simulink model "SARADC"  (R2024a)
settings: Solver=VariableStepAuto  StartTime=0.0  StopTime=10.0  RelTol=1e-3
undefined symbols (not defined in the file): bs2, bs3, bs4, bs5, thnoise_samp
settings Model: Creator=sjtu  LastModifiedBy=sjtu

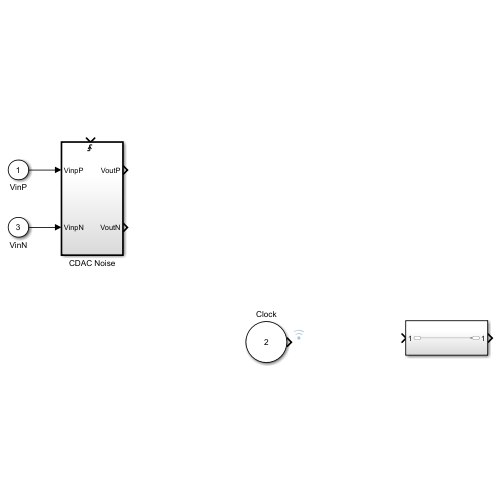
[thumbnail: Simulink's stored preview of the top-level diagram]
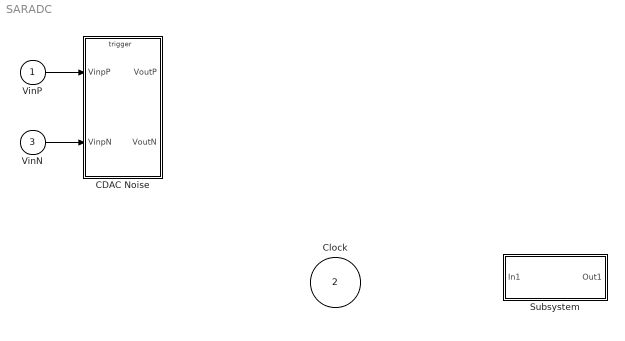
== system SARADC ==
  VinP : Inport
  Clock : Inport  Port=2
  VinN : Inport  Port=3
  CDAC Noise : Subsystem  TreatAsAtomicUnit=on
  Subsystem : Subsystem
  wires:
  VinN/1 -> CDAC Noise/2(VinpN)
  VinP/1 -> CDAC Noise/1(VinpP)

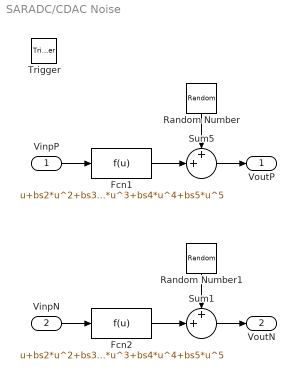
== system SARADC/CDAC Noise ==
  VinpP : Inport
  VinpN : Inport  Port=2
  Trigger : TriggerPort  VariantControl=Variant
  Fcn1 : Fcn  Expr=u+bs2*u^2+bs3*u^3+bs4*u^4+bs5*u^5
  Fcn2 : Fcn  Expr=u+bs2*u^2+bs3*u^3+bs4*u^4+bs5*u^5
  Random Number : RandomNumber  Variance=thnoise_samp  Seed=1
  Random Number1 : RandomNumber  Variance=thnoise_samp  Seed=2
  Sum1 : Sum  Inputs=++|  SaturateOnIntegerOverflow=on
  Sum5 : Sum  Inputs=++|  SaturateOnIntegerOverflow=on
  VoutP : Outport
  VoutN : Outport  Port=2
  wires:
  VinpP/1 -> Fcn1/1
  VinpN/1 -> Fcn2/1
  Fcn1/1 -> Sum5/2
  Fcn2/1 -> Sum1/2
  Sum5/1 -> VoutP/1
  Sum1/1 -> VoutN/1
  Random Number/1 -> Sum5/1
  Random Number1/1 -> Sum1/1

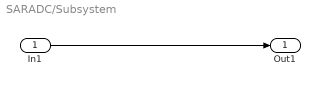
== system SARADC/Subsystem ==
  In1 : Inport
  Out1 : Outport
  wires:
  In1/1 -> Out1/1
